simulink model "stateflow_function"  (R2022b)
settings: Solver=ode1  StartTime=0.0  StopTime=inf  FixedStep=0.001  RelTol=1e-3
settings Model: Creator=user  LastModifiedBy=user

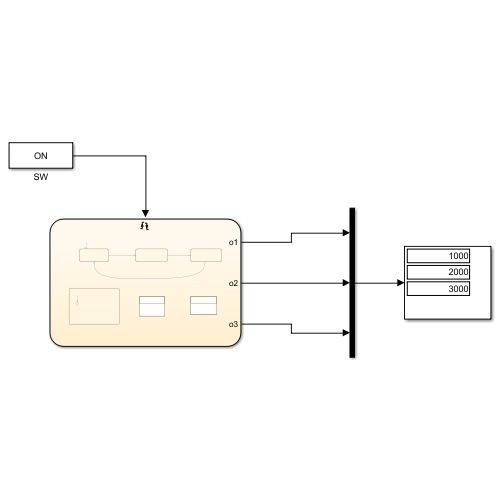
[thumbnail: Simulink's stored preview of the top-level diagram]
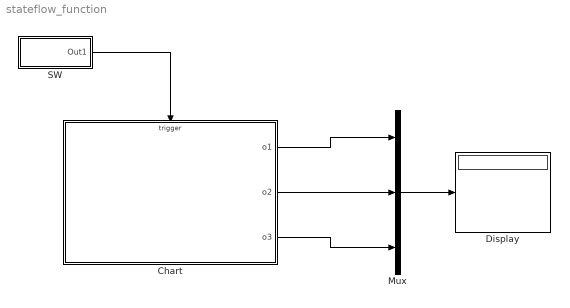
== system stateflow_function ==
  Chart : Stateflow chart  TreatAsAtomicUnit=on
  Display : Display
  Mux : Mux  Inputs=3
  SW : Subsystem  StartFcn=|  mask{str=ON}
      | set_param(gcb, 'str', 'OFF');
      | set_param([gcb '/Constant'], 'Value', '0');
      mask prompts: str "Display name:"
      settings: OpenFcn=|
      | old_val = get_param([gcb '/Constant'], 'Value');
      | 
      | switch old_val
      | case '0'
      |     set_param(gcb, 'str', 'ON');
      |     set_param([gcb '/Constant'], 'Value', '1');
      | 
      | case '1'
      |     set_param(gcb, 'str', 'OFF');
      |     set_param([gcb '/Constant'], 'Value', '0');
      | 
      | otherwise
      |     set_param(gcb, 'str', 'ON');
      |     set_param([gcb '/Constant'], 'Value', '0');
      | 
      | end
      mask DialogControl ParameterGroupVar Prompt: 파라미터
      mask Display: disp(get_param(gcb,'str'));
  wires:
  SW/1(Out1) -> Chart/Trigger
  Chart/1(o1) -> Mux/1
  Chart/2(o2) -> Mux/2
  Chart/3(o3) -> Mux/3
  Mux/1 -> Display/1

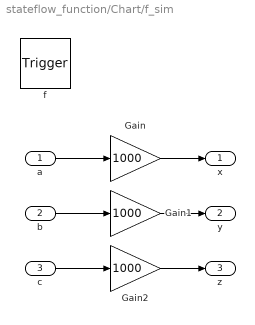
== system stateflow_function/Chart/f_sim ==
  a : Inport  OutDataTypeStr=double  PortDimensions=1
  b : Inport  Port=2  OutDataTypeStr=double  PortDimensions=1
  c : Inport  Port=3  OutDataTypeStr=double  PortDimensions=1
  f : TriggerPort  TriggerType=function-call  VariantControl=(inherit)
      settings: CopyFcn=Stateflow.SLINSF.SimulinkMan.removeBlockPreDeleteFcn  PreDeleteFcn=Stateflow.SLINSF.SimulinkMan.unsafePredeleteFcn
  Gain : Gain  Gain=1000
  Gain1 : Gain  Gain=1000
  Gain2 : Gain  Gain=1000
  x : Outport
  y : Outport  Port=2
  z : Outport  Port=3
  wires:
  a/1 -> Gain/1
  Gain/1 -> x/1
  b/1 -> Gain1/1
  Gain1/1 -> y/1
  c/1 -> Gain2/1
  Gain2/1 -> z/1

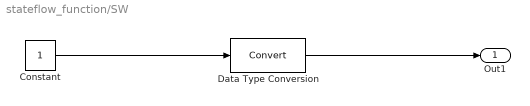
== system stateflow_function/SW ==
  Constant : Constant
  Data Type Conversion : DataTypeConversion  SaturateOnIntegerOverflow=off  RndMeth=Floor
  Out1 : Outport
  wires:
  Data Type Conversion/1 -> Out1/1
  Constant/1 -> Data Type Conversion/1

== stateflow chart stateflow_function/Chart ==
  settings: executeAtInitialization=1
  state a
    en:
    [o1,o2,o3] = f_sf(1,2,3);
  state b
    en:
    [o1,o2,o3] = f_mat(1,2,3);
  state c
    en:
    [o1,o2,o3] = f_sim(1,2,3);
  state [x,y,z] = f_sf(a,b,c) [function]
    (default) -> (junction 6) : {
        | x = 10*a;
        | y = 10*b;
        | z = 10*c;
        | }
  state [x,y,z] = f_sim(a,b,c) [function]
  (default) -> a
  a -> b : E
  b -> c : E
  c -> a : E
  data: a function_input; b function_input; c function_input; x function_output; y function_output; z function_output; a function_input; b function_input; c function_input; x function_output; y function_output; z function_output; a function_input double size=1; b function_input double size=1; c function_input double size=1; x function_output; y function_output; z function_output; o1 output; o2 output; o3 output
  events: E input EITHER_EDGE_EVENT
  function [x,y,z] = f_mat(a,b,c):
    | function [x,y,z] = f_mat(a,b,c)
    | x = 100*a;
    | y = 100*b;
    | z = 100*c;
    | end
